simulink subsystem "LimitedSlipDifferentialSSC"  (R2025a)
settings: Solver=VariableStepAuto  StartTime=0.0  StopTime=10.0  RelTol=1e-3
undefined symbols (not defined in the file): AxlFL, AxlFR, PlntDiffrntlAxl1Damp, PlntDiffrntlCarrDamp, PlntDiffrntlEff, PlntDiffrntlPwrThresh, PlntDriveshftStiff
libraries: sdl_lib x3, fl_lib x2
settings Model: ModifiedByFormat=The MathWorks, Inc.  Creator=The MathWorks, Inc.  LastModifiedBy=The MathWorks, Inc.
settings OptimizationCC: ReuseModelBlockBuffer=off
settings RTWCC: GPUComputeCapability=3.5

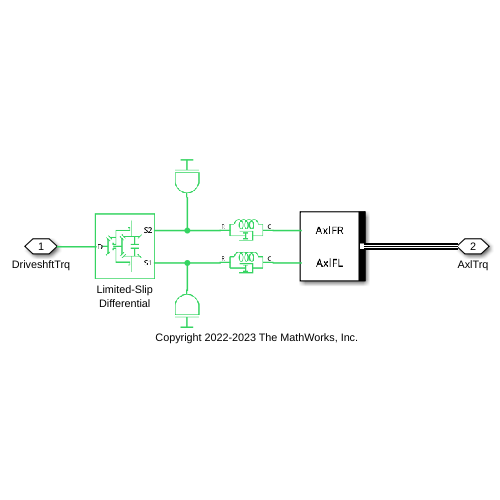
[thumbnail: Simulink's stored preview of the top-level diagram]
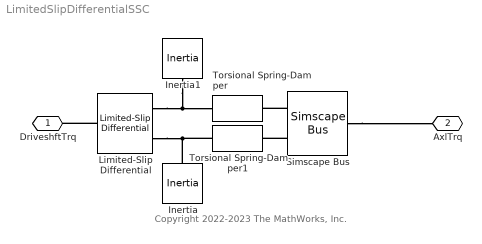
== system LimitedSlipDifferentialSSC ==
  note: Copyright 2022-2023 The MathWorks, Inc.
  Inertia : fl_lib/Mechanical/Rotational Elements/Inertia  inertia=PlntDiffrntlAxl1Inertia kg*m^2  num_ports=foundation.enum.numPorts2.one  w_specify=off  w_priority=High  w=0 rad/s  w_nominal_specify=off  w_nominal_value=1  w_nominal_unit=rad/s  t_specify=off  t_priority=None  t=0 N*m  t_nominal_specify=off  t_nominal_value=1  t_nominal_unit=N*m
      settings: SourceProductName=Foundation Library
  Inertia1 : fl_lib/Mechanical/Rotational Elements/Inertia  inertia=PlntDiffrntlAxl2Inertia kg*m^2  num_ports=foundation.enum.numPorts2.one  w_specify=off  w_priority=High  w=0 rad/s  w_nominal_specify=off  w_nominal_value=1  w_nominal_unit=rad/s  t_specify=off  t_priority=None  t=0 N*m  t_nominal_specify=off  t_nominal_value=1  t_nominal_unit=N*m
      settings: SourceProductName=Foundation Library
  Limited-Slip Differential : sdl_lib/Gears/Limited-Slip Differential  driveshaft_location=sdl.enum.differential_orientation.right  cd_ratio=PlntDiffrntlRatio  friction_model=sdl.enum.gear_friction.constant  efficiency=[PlntDiffrntlEff PlntDiffrntlEff]  temperature_TLU=[280, 300, 320] K  efficiency_ss_TLU=[.95, .9, .85]  efficiency_cd_TLU=[.95, .9, .85]  pwr_thr=[PlntDiffrntlPwrThresh, PlntDiffrntlPwrThresh] W  mu_visc=[PlntDiffrntlCarrDamp PlntDiffrntlAxl1Damp] N*m*s/rad  model_inertia=simscape.enum.onoff.off  sun_inertia=1e-10 kg*m^2  sun_radius=0.01 m  carrier_inertia=PlntDiffrntlCarrInertia kg*m^2  planet_inertia=PlntDiffrntlAxl1Inertia kg*m^2  planet_mass=1e-10 kg  nS=PlntDiffrntlCltchNumDisk  r_eff=PlntDiffrntlCltchRadius m  force_preload=PlntDiffrntlCltchPreloadForce N  mu_static=PlntDiffrntlCltchStatFric  mu_static_vector=[.4, .38, .36]  mu_w_vector=PlntDiffrntlCltchSpdVect rad/s  mu_coulomb_vector=PlntDiffrntlCltchFricVect  mu_coulomb_matrix=[.34, .32, .3; .3, .28, .25; .25, .2, .15]  mu_interp_method=simscape.enum.interpolation.linear  mu_extrap_method=simscape.enum.extrapolation.linear  w_tol=PlntDiffrntlCltchVelTol rad/s  initial_state_locked=sdl.enum.initial_lock.unlocked  thermal_mass=50 J/K  T_init=300 K
      settings: SourceProductName=Driveline  InternalSimscapePortConfiguration="{\"Bottom\":[],\"Left\":[{\"id\":\"D\",\"label\":\"D\",\"type\":\"foundation.mechanical.rotational.rotational\"}],\"Right\":[{\"id\":\"S1\",\"label\":\"S1\",\"type\":\"foundation.mechanical.rotational.rotational\"},{\"id\":\"S2\",\"label\":\"S2\",\"type\":\"foundation.mechanical.rotational.rotational\"}],\"Top\":[]}"
  Simscape Bus : SimscapeBus  HierarchyStrings=AxlFR;AxlFL
  Torsional Spring-Damper : sdl_lib/Couplings & Drives/Torsional Spring-Damper  k=PlntDriveshftStiff N*m/rad  mu_visc=PlntDriveshftDamp N*m*s/rad  trq_coulomb=0 N*m  static_kinetic_ratio=1.1  w_tol=0.001 rad/s  model_hardstop=sdl.enum.hardStopOffOn.off  upper_bound=10 deg  lower_bound=-10 deg  hardstop_model=simscape.enum.hardstop.smooth  k_endstop=1e6 N*m/rad  D_endstop=10 N*m*s/rad  transition=0.001 rad  coeff_rest=0.7  w_tol_hardstop=0.1 rad/s  trq_tol=0.001 N*m  x0=0 deg
      settings: SourceProductName=Driveline  InternalSimscapePortConfiguration="{\"Bottom\":[],\"Left\":[{\"id\":\"R\",\"label\":\"R\",\"type\":\"foundation.mechanical.rotational.rotational\"}],\"Right\":[{\"id\":\"C\",\"label\":\"C\",\"type\":\"foundation.mechanical.rotational.rotational\"}],\"Top\":[]}"
  Torsional Spring-Damper1 : sdl_lib/Couplings & Drives/Torsional Spring-Damper  k=PlntDriveshftStiff N*m/rad  mu_visc=PlntDriveshftDamp N*m*s/rad  trq_coulomb=0 N*m  static_kinetic_ratio=1.1  w_tol=0.001 rad/s  model_hardstop=sdl.enum.hardStopOffOn.off  upper_bound=10 deg  lower_bound=-10 deg  hardstop_model=simscape.enum.hardstop.smooth  k_endstop=1e6 N*m/rad  D_endstop=10 N*m*s/rad  transition=0.001 rad  coeff_rest=0.7  w_tol_hardstop=0.1 rad/s  trq_tol=0.001 N*m  x0=0 deg
      settings: SourceProductName=Driveline  InternalSimscapePortConfiguration="{\"Bottom\":[],\"Left\":[{\"id\":\"R\",\"label\":\"R\",\"type\":\"foundation.mechanical.rotational.rotational\"}],\"Right\":[{\"id\":\"C\",\"label\":\"C\",\"type\":\"foundation.mechanical.rotational.rotational\"}],\"Top\":[]}"
  DriveshftTrq : PMIOPort  Side=Left
  AxlTrq : PMIOPort  Port=2  Side=Right
  connections:
  Limited-Slip Differential/LConn1 -- DriveshftTrq/RConn1
  Simscape Bus/RConn1 -- AxlTrq/RConn1
  Inertia1/LConn1 -- Limited-Slip Differential/RConn2 -- Torsional Spring-Damper/LConn1
  Inertia/LConn1 -- Limited-Slip Differential/RConn1 -- Torsional Spring-Damper1/LConn1
  Simscape Bus/LConn1 -- Torsional Spring-Damper/RConn1
  Simscape Bus/LConn2 -- Torsional Spring-Damper1/RConn1
